simulink model "DecoderBinary2Dec"  (R2014a)
settings: Solver=FixedStepDiscrete  StartTime=0.0  StopTime=2  FixedStep=1  RelTol=1e-3
libraries: commutil2 x1
settings Model: Creator=The MathWorks Inc.  LastModifiedBy=Tanvir
settings DataIOCC: SignalLoggingSaveFormat=ModelDataLogs
settings OptimizationCC: ExpressionDepthLimit=2147483647
settings DebuggingCC: UnderspecifiedInitializationDetection=Classic  FcnCallInpInsideContextMsg=UseLocalSettings  StateNameClashWarn=warning
settings RTWCC: ProcessScript=grt_make_rtw_hook
settings GRTTargetCC: CombineOutputUpdateFcns=off  GRTInterface=on

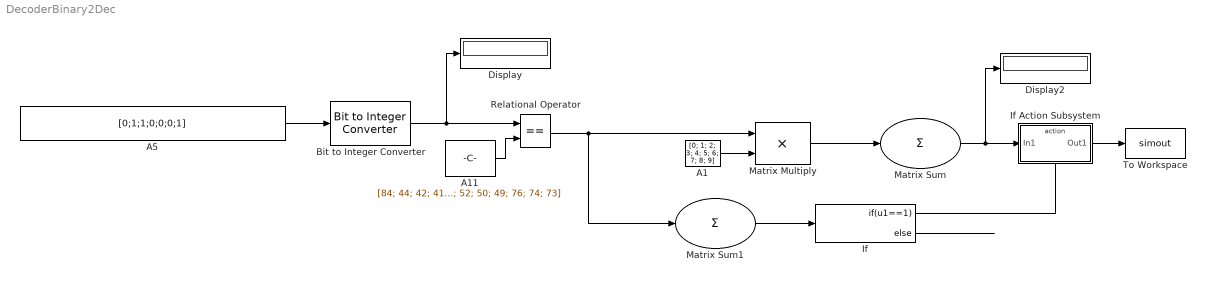
== system DecoderBinary2Dec ==
  A1 : Constant  Value=[0; 1; 2; 3; 4; 5; 6; 7; 8; 9]
  A11 : Constant  Value=[84; 44; 42; 41; 52; 50; 49; 76; 74; 73]
  A5 : Constant  Value=[0;1;1;0;0;0;1]
  Bit to Integer Converter : commutil2/Bit to Integer Converter  nbits=7  bitOrder=MSB first  signedOutputValues=Unsigned  outDtype=Inherit via internal rule  outDtypeSigned=Inherit via internal rule
  Display : Display
  Display2 : Display
  If : If  IfExpression=u1==1
  If Action Subsystem : Subsystem  TreatAsAtomicUnit=on
  Matrix Sum : Sum  Inputs=+  OutDataTypeStr=double
  Matrix Sum1 : Sum  Inputs=+  OutDataTypeStr=double
  Matrix Multiply : Product
  Relational Operator : RelationalOperator  Operator===  OutDataTypeStr=boolean
  To Workspace : ToWorkspace  VariableName=simout  SaveFormat=Timeseries  SampleTime=-1
  wires:
  A5/1 -> Bit to Integer Converter/1
  Bit to Integer Converter/1 -> Display/1, Relational Operator/1
  Relational Operator/1 -> Matrix Multiply/1, Matrix Sum1/1
  A11/1 -> Relational Operator/2
  A1/1 -> Matrix Multiply/2
  If/1 -> If Action Subsystem/Action
  Matrix Sum1/1 -> If/1
  If Action Subsystem/1(Out1) -> To Workspace/1
  Matrix Sum/1 -> Display2/1, If Action Subsystem/1(In1)
  Matrix Multiply/1 -> Matrix Sum/1
  If/2 -> ?

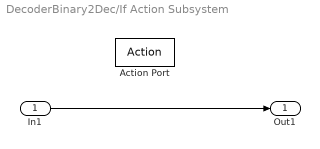
== system DecoderBinary2Dec/If Action Subsystem ==
  In1 : Inport
  Action Port : ActionPort  ActionType=then
  Out1 : Outport
  wires:
  In1/1 -> Out1/1
